simulink model "state_space_control_pendulum_cart_with_observer"  (R2021b)
settings: Solver=VariableStepAuto  StartTime=0.0  StopTime=10.0  RelTol=1e-3
values from neighbouring files (symbols this model uses):
  A = [0       0             1           0 ... (first row only)    [task_1.m]
  Ad = sys_d.a    [task_1.m]
  B = [0;0;1/mc;1/(L*mc)]    [task_1.m]
  Bd = sys_d.b    [task_1.m]
  Cd = sys_d.c    [task_1.m]
  K_d = acker(Ad,Bd,d_poles_D)    [task_1.m]
  ob = acker(Ad',Cd',d_poles_D)    [task_1.m]
  Ts = 0.1    [task_1.m]
  x0 = [0;5*pi/180;0;0]    [task_1.m]
settings Model: Creator=ANUBHAV  LastModifiedBy=ANUBHAV

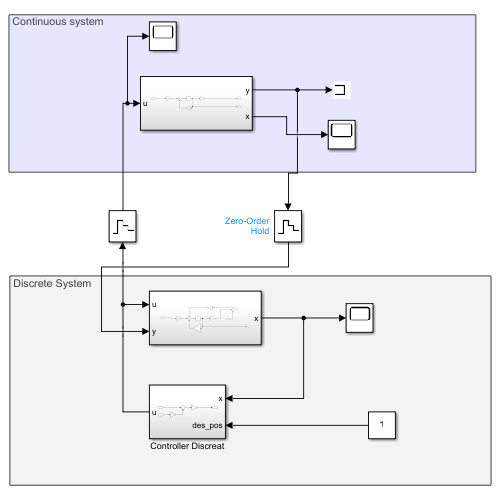
[thumbnail: Simulink's stored preview of the top-level diagram]
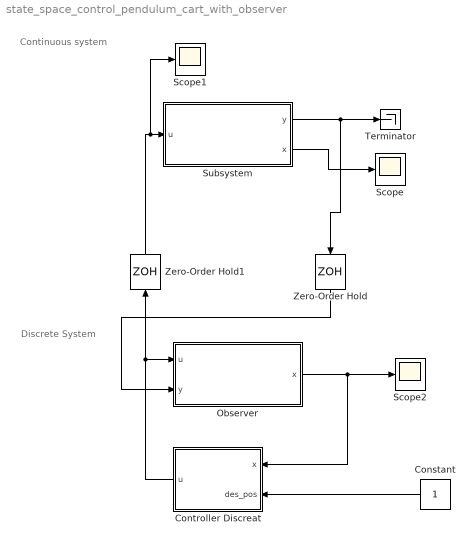
== system state_space_control_pendulum_cart_with_observer ==
  note: Continuous system
  note: Discrete System
  Constant : Constant
  Controller Discreat : Subsystem
  Observer : Subsystem
  Scope : Scope
  Scope1 : Scope
  Scope2 : Scope
  Subsystem : Subsystem
  Terminator : Terminator
  Zero-Order Hold : ZeroOrderHold  SampleTime=Ts
  Zero-Order Hold1 : ZeroOrderHold  SampleTime=Ts
  wires:
  Constant/1 -> Controller Discreat/2(des_pos)
  Subsystem/2(x) -> Scope/1
  Zero-Order Hold1/1 -> Scope1/1, Subsystem/1(u)
  Controller Discreat/1(u) -> Zero-Order Hold1/1, Observer/1(u)
  Subsystem/1(y) -> Terminator/1, Zero-Order Hold/1
  Zero-Order Hold/1 -> Observer/2(y)
  Observer/1(x) -> Controller Discreat/1(x), Scope2/1

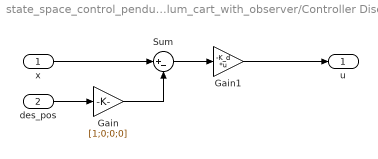
== system state_space_control_pendulum_cart_with_observer/Controller Discreat ==
  x : Inport
  des_pos : Inport  Port=2
  Gain : Gain  Gain=[1;0;0;0]
  Gain1 : Gain  Gain=-K_d  Multiplication=Matrix(K*u) (u vector)
  Sum : Sum  Inputs=|+-
  u : Outport
  wires:
  Gain1/1 -> u/1
  x/1 -> Sum/1
  Sum/1 -> Gain1/1
  des_pos/1 -> Gain/1
  Gain/1 -> Sum/2

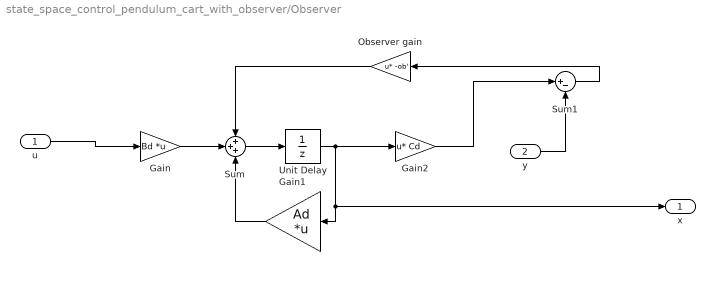
== system state_space_control_pendulum_cart_with_observer/Observer ==
  u : Inport
  y : Inport  Port=2
  Gain : Gain  Gain=Bd  Multiplication=Matrix(K*u)
  Gain1 : Gain  Gain=Ad  Multiplication=Matrix(K*u) (u vector)
  Gain2 : Gain  Gain=Cd  Multiplication=Matrix(u*K)
  Observer gain : Gain  Gain=-ob'  Multiplication=Matrix(u*K)
  Sum : Sum  Inputs=+++
  Sum1 : Sum  Inputs=|+-
  Unit Delay : UnitDelay  InitialCondition=x0*0  SampleTime=-1  HasFrameUpgradeWarning=on
  x : Outport
  wires:
  u/1 -> Gain/1
  Gain2/1 -> Sum1/1
  Unit Delay/1 -> Gain1/1, x/1, Gain2/1
  Sum/1 -> Unit Delay/1
  y/1 -> Sum1/2
  Sum1/1 -> Observer gain/1
  Gain/1 -> Sum/2
  Gain1/1 -> Sum/3
  Observer gain/1 -> Sum/1

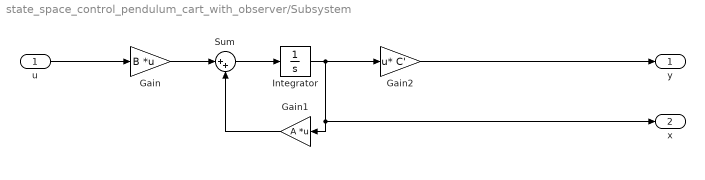
== system state_space_control_pendulum_cart_with_observer/Subsystem ==
  u : Inport
  Gain : Gain  Gain=B  Multiplication=Matrix(K*u)
  Gain1 : Gain  Gain=A  Multiplication=Matrix(K*u) (u vector)
  Gain2 : Gain  Gain=C'  Multiplication=Matrix(u*K)
  Integrator : Integrator  InitialCondition=x0
  Sum : Sum  Inputs=|++
  y : Outport
  x : Outport  Port=2
  wires:
  Gain1/1 -> Sum/2
  Integrator/1 -> Gain2/1, x/1, Gain1/1
  Gain2/1 -> y/1
  Gain/1 -> Sum/1
  Sum/1 -> Integrator/1
  u/1 -> Gain/1
